simulink model "pend_sim_euler"  (R2013a)
settings: Solver=ode1  StartTime=0.0  StopTime=(length(control)-1)*dt  FixedStep=dt  RelTol=1e-3
StopFcn:
  | hf = findall(0,'Name','XY Graph'); %handle to figure window
  | ha = findall(hf,'Type','axes'); %handle to axis
  | set(ha,'XGrid','on','YGrid','on') % trun the grid on
  | set(ha,'XTick',-pi:pi/4:pi,'XTickLabel',{'-pi','-3pi/4','-pi/2','-pi/4','0','pi/4','pi/2','3pi/4','pi'});
values from neighbouring files (symbols this model uses):
  b = 0.1    [RRT_pend.m]    (also in RRT_pend_codegen.m; RRT_pend_fromC.m; RRT_pend_novisuals.m)
  g = 9.8    [RRT_pend.m]    (also in RRT_pend_codegen.m; RRT_pend_fromC.m; RRT_pend_novisuals.m)
  l = 1    [RRT_pend.m]    (also in RRT_pend_codegen.m; RRT_pend_fromC.m; RRT_pend_novisuals.m)
  m = 1    [RRT_pend.m]    (also in RRT_pend_codegen.m; RRT_pend_fromC.m; RRT_pend_novisuals.m)
  N = 50000    [RRT_pend.m]    (also in RRT_pend_codegen.m = 20000; RRT_pend_novisuals.m)
  theta_0 = -pi/2    (= -1.57079632679)    [RRT_pend.m]    (also in RRT_pend_fromC.m; RRT_pend_novisuals.m)
libraries: mblibv1 x5, simulink x1
settings Model: Creator=nightling  LastModifiedBy=nightling
settings SimMechanicsCC: VisOnUpdateDiagram=on  VisDuringSimulation=on

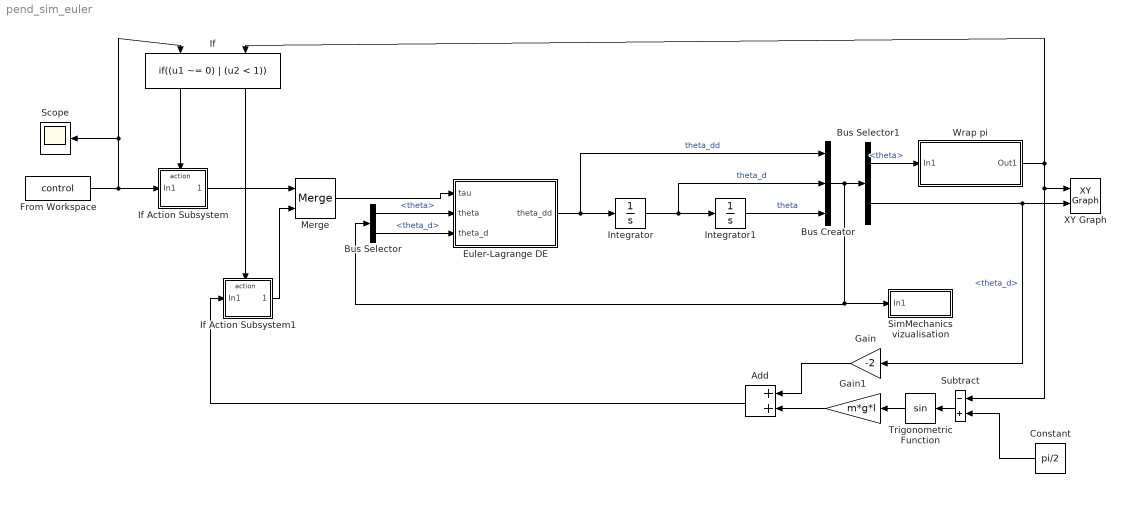
== system pend_sim_euler ==
  Add : Sum
  Bus Creator : BusCreator  Inputs=3
  Bus Selector : BusSelector  OutputSignals=theta,theta_d
  Bus Selector1 : BusSelector  OutputSignals=theta,theta_d
  Constant : Constant  Value=pi/2
  Euler-Lagrange DE : Subsystem
  From Workspace : FromWorkspace  VariableName=control  OutDataTypeStr=double  SampleTime=0  Interpolate=off  OutputAfterFinalValue=Setting to zero
  Gain : Gain  Gain=-2
  Gain1 : Gain  Gain=m*g*l
  If : If  NumInputs=2  IfExpression=(u1 ~= 0) | (u2 < 1)
  If Action Subsystem : Subsystem  TreatAsAtomicUnit=on
  If Action Subsystem1 : Subsystem  TreatAsAtomicUnit=on
  Integrator : Integrator
  Integrator1 : Integrator  InitialCondition=theta_0
  Merge : Merge
  Scope : Scope
      settings: YMax=10
  SimMechanics vizualisation : Subsystem
  Subtract : Sum  Inputs=-+
  Trigonometric Function : Trigonometry
  Wrap pi : Subsystem
  XY Graph : simulink/Sinks/XY Graph  xmin=-pi  xmax=pi  ymin=-10  ymax=10  st=-1
  wires:
  Euler-Lagrange DE/1(theta_dd) -> Bus Creator/1, Integrator/1  "theta_dd"
  Integrator/1 -> Bus Creator/2, Integrator1/1  "theta_d"
  Integrator1/1 -> Bus Creator/3  "theta"
  Bus Creator/1 -> SimMechanics vizualisation/1(In1), Bus Selector/1, Bus Selector1/1
  Bus Selector/1 -> Euler-Lagrange DE/2(theta)  "<theta>"
  Bus Selector/2 -> Euler-Lagrange DE/3(theta_d)  "<theta_d>"
  Merge/1 -> Euler-Lagrange DE/1(tau)
  Bus Selector1/2 -> Gain/1, XY Graph/2  "<theta_d>"
  Bus Selector1/1 -> Wrap pi/1(In1)  "<theta>"
  Wrap pi/1(Out1) -> Subtract/1, XY Graph/1, If/2
  Trigonometric Function/1 -> Gain1/1
  Constant/1 -> Subtract/2
  Subtract/1 -> Trigonometric Function/1
  If/1 -> If Action Subsystem/Action
  If/2 -> If Action Subsystem1/Action
  From Workspace/1 -> If/1, Scope/1, If Action Subsystem/1(In1)
  If Action Subsystem/1(Out1) -> Merge/1
  If Action Subsystem1/1(Out1) -> Merge/2
  Gain1/1 -> Add/2
  Gain/1 -> Add/1
  Add/1 -> If Action Subsystem1/1(In1)

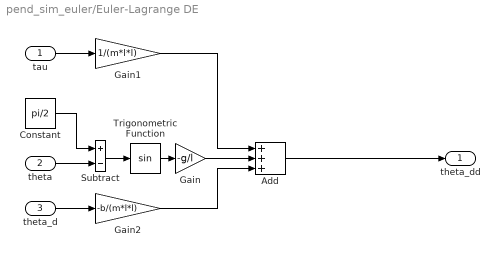
== system pend_sim_euler/Euler-Lagrange DE ==
  tau : Inport
  theta : Inport  Port=2
  theta_d : Inport  Port=3
  Add : Sum  Inputs=+++
  Constant : Constant  Value=pi/2
  Gain : Gain  Gain=-g/l
  Gain1 : Gain  Gain=1/(m*l*l)
  Gain2 : Gain  Gain=-b/(m*l*l)
  Subtract : Sum  Inputs=+-
  Trigonometric Function : Trigonometry
  theta_dd : Outport
  wires:
  Trigonometric Function/1 -> Gain/1
  theta_d/1 -> Gain2/1
  tau/1 -> Gain1/1
  Gain/1 -> Add/2
  Gain2/1 -> Add/3
  Gain1/1 -> Add/1
  theta/1 -> Subtract/2
  Constant/1 -> Subtract/1
  Subtract/1 -> Trigonometric Function/1
  Add/1 -> theta_dd/1

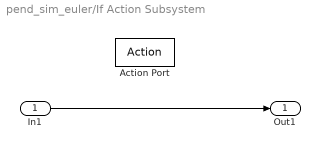
== system pend_sim_euler/If Action Subsystem ==
  In1 : Inport
  Action Port : ActionPort  ActionType=then
  Out1 : Outport
  wires:
  In1/1 -> Out1/1

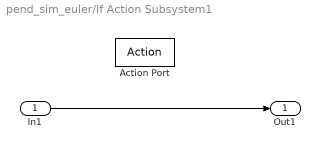
== system pend_sim_euler/If Action Subsystem1 ==
  In1 : Inport
  Action Port : ActionPort  ActionType=else
  Out1 : Outport
  wires:
  In1/1 -> Out1/1

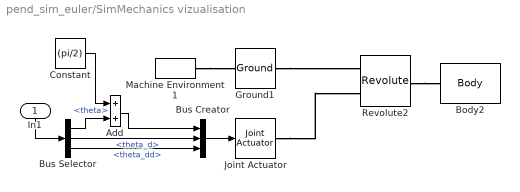
== system pend_sim_euler/SimMechanics vizualisation ==
  In1 : Inport
  Add : Sum
  Body2 : mblibv1/Bodies/Body  LConnTagsString=CS1  RConnTagsString=CS2  UpdateFromCAD=off  DialogClass=MechanicalBodyBlock  Mass=m  MassUnits=kg  InertiaUnits=kg*m^2  Inertia=zeros(3)  Shape=Cylinder  ShapeDims=[1 1]  ShapeUnits=m  ShapeUse=false  Density=1  DensityUnits=kg/m^3  DensityUse=false  GraphicsMode=MACHINE_DEFAULT  BodyColorSelMode=COLORPALETTE  BodyColor=[0.043137 0.51765 0.78039]  AttachedToCS=CG  CG=Left$CG$[0 -l/2 0]$CS1$CS1$m$[0 0 0]$Euler X-Y-Z$deg$WORLD$false$none  WorkingFrames=Left$CS1$[0 0 0]$Adjoining$Adjoining$m$[0 0 0]$Euler X-Y-Z$deg$WORLD$true$none#Right$CS2$[0 -l 0]$CS1$CS1$m$[0 0 0]$Euler X-Y-Z$deg$WORLD$true$none  CGPos=[0 -l/2 0]  CGRot=[0 0 0]  CS0Pos=[]  CS0Rot=[]  CS1Pos=[0 0 0]  CS1Rot=[0 0 0]  CS2Pos=[0 -l 0]  CS2Rot=[0 0 0]  CS3Pos=[]  CS3Rot=[]  CS4Pos=[]  CS4Rot=[]  CS5Pos=[]  CS5Rot=[]  CS6Pos=[]  CS6Rot=[]  CS7Pos=[]  CS7Rot=[]  CS8Pos=[]  CS8Rot=[]  CS9Pos=[]  CS9Rot=[]  CS10Pos=[]  CS10Rot=[]  CS11Pos=[]  CS11Rot=[]  CS12Pos=[]  CS12Rot=[]  CS13Pos=[]  CS13Rot=[]  CS14Pos=[]  CS14Rot=[]  CS15Pos=[]  CS15Rot=[]  CS16Pos=[]  CS16Rot=[]  CS17Pos=[]  CS17Rot=[]  CS18Pos=[]  CS18Rot=[]  CS19Pos=[]  CS19Rot=[]  CS20Pos=[]  CS20Rot=[]
  Bus Creator : BusCreator  Inputs=3
  Bus Selector : BusSelector  OutputSignals=theta,theta_d,theta_dd
  Constant : Constant  Value=(pi/2)
  Ground1 : mblibv1/Bodies/Ground  UpdateFromCAD=off  LeftPortType=env  RightPortType=workingframe  PhysicalDomain=Mechanical  DialogClass=GroundBlock  CoordPosition=[1 0 0]  CoordPositionUnits=m  StateVectorMgrId=0  MachineId=[1 0]  ShowEnvPort=on
  Joint Actuator : mblibv1/Sensors &  Actuators/Joint Actuator  UpdateFromCAD=off  PhysicalDomain=Mechanical  PortType=blob  ActuationStyle=Motion  AngleUnits=rad  ArcVelocityUnits=rad/s  ArcAccelerationUnits=rad/s^2  CoordPositionUnits=m  VelocityUnits=m/s  AccelerationUnits=m/s^2  ForceUnits=N  TorqueUnits=N*m  ActiveIO=on  Width=3  DialogClass=MechanicalActuatorBlock  Primitive=R1  ReferenceFrame=Absolute (World)
  Machine Environment1 : mblibv1/Bodies/Machine Environment  PortType=env  PhysicalDomain=Mechanical  DialogTemplateClass=MECH.MachineEnvironment  SyncWhenCopied=off  Gravity=[0 -9.8 0]  GravityUnits=m/s^2  GravityAsSignal=off  Dimensionality=Auto-detect  AnalysisType=Forward dynamics  LinearAssemblyTolerance=1e-3  LinearAssemblyToleranceUnits=m  AngularAssemblyTolerance=1e-3  AngularAssemblyToleranceUnits=rad  ConstraintSolverType=Stabilizing  ConstraintRelTolerance=1e-4  ConstraintAbsTolerance=1e-4  UseRobustSingularityHandling=off  RedundancyAnalysisToleranceType=Automatically select tolerance  RedundancyAnalysisTolerance=1e-14  StatePerturbationType=Fixed  PerturbationSize=1e-5  VisualizeMachine=on  BodyVisualizationType=Use model default body geometries  BodyColorSelMode=Use model default  DefaultBodyColor=[1 0 0]
  Revolute2 : mblibv1/Joints/Revolute  LConnTagsString=__newl0|SA1  RConnTagsString=__newr0  UpdateFromCAD=off  NumSAPorts=1  CutJoint=off  MarkAsCut=off  Primitives=prismatic  PrimitiveProps=R1$World$[0 0 1]$revolute  DialogClass=JointBlock  R1Axis=[0 0 1]
  wires:
  Bus Creator/1 -> Joint Actuator/1
  In1/1 -> Bus Selector/1
  Bus Selector/1 -> Add/2  "<theta>"
  Add/1 -> Bus Creator/1
  Bus Selector/2 -> Bus Creator/2  "<theta_d>"
  Bus Selector/3 -> Bus Creator/3  "<theta_dd>"
  Constant/1 -> Add/1
  connections:
  Revolute2/RConn1 -- Body2/LConn1
  Machine Environment1/RConn1 -- Ground1/LConn1
  Ground1/RConn1 -- Revolute2/LConn1
  Joint Actuator/RConn1 -- Revolute2/LConn2

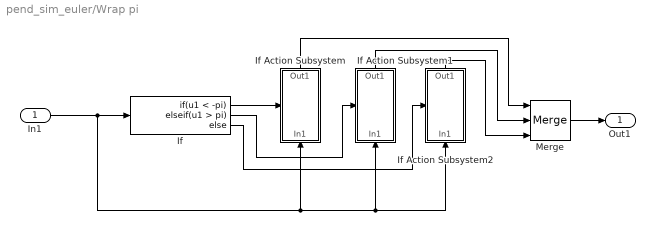
== system pend_sim_euler/Wrap pi ==
  In1 : Inport
  If : If  IfExpression=u1 < -pi  ElseIfExpressions=u1 > pi
  If Action Subsystem : Subsystem  TreatAsAtomicUnit=on
  If Action Subsystem1 : Subsystem  TreatAsAtomicUnit=on
  If Action Subsystem2 : Subsystem  TreatAsAtomicUnit=on
  Merge : Merge  Inputs=3
  Out1 : Outport
  wires:
  If/1 -> If Action Subsystem/Action
  In1/1 -> If Action Subsystem2/1(In1), If Action Subsystem1/1(In1), If Action Subsystem/1(In1), If/1
  If Action Subsystem/1(Out1) -> Merge/1
  If/2 -> If Action Subsystem1/Action
  If Action Subsystem1/1(Out1) -> Merge/2
  If Action Subsystem2/1(Out1) -> Merge/3
  If/3 -> If Action Subsystem2/Action
  Merge/1 -> Out1/1

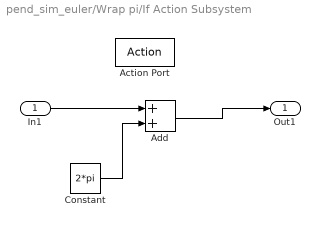
== system pend_sim_euler/Wrap pi/If Action Subsystem ==
  In1 : Inport
  Action Port : ActionPort  ActionType=then
  Add : Sum
  Constant : Constant  Value=2*pi
  Out1 : Outport
  wires:
  In1/1 -> Add/1
  Constant/1 -> Add/2
  Add/1 -> Out1/1

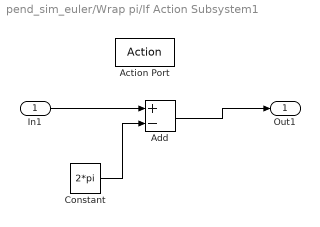
== system pend_sim_euler/Wrap pi/If Action Subsystem1 ==
  In1 : Inport
  Action Port : ActionPort  ActionType=elseif
  Add : Sum  Inputs=+-
  Constant : Constant  Value=2*pi
  Out1 : Outport
  wires:
  In1/1 -> Add/1
  Constant/1 -> Add/2
  Add/1 -> Out1/1

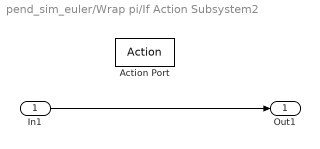
== system pend_sim_euler/Wrap pi/If Action Subsystem2 ==
  In1 : Inport
  Action Port : ActionPort  ActionType=else
  Out1 : Outport
  wires:
  In1/1 -> Out1/1
